simulink model "sampleModel206"  (R2021b)
settings: Solver=VariableStepAuto  StartTime=0.0  StopTime=10.0  RelTol=1e-3
libraries: simulink x9, slpidlib x1
settings Model: Creator=user  LastModifiedBy=user

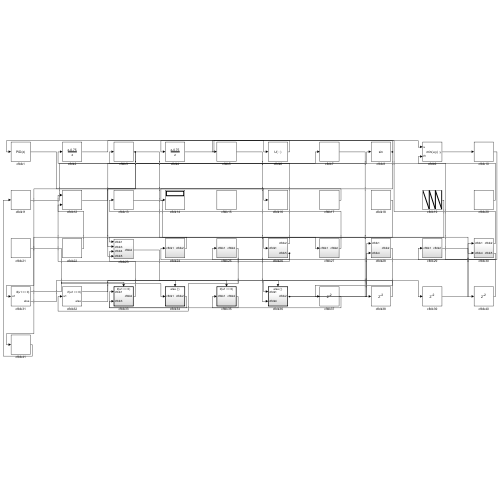
[thumbnail: Simulink's stored preview of the top-level diagram]
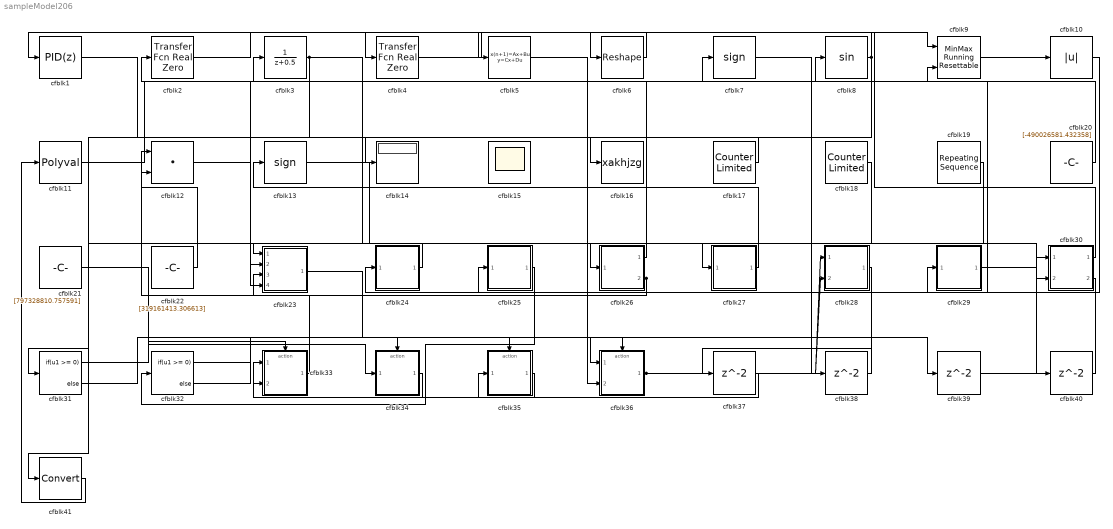
== system sampleModel206 ==
  cfblk1 : slpidlib/PID Controller  Controller=PID  Form=Parallel  TimeDomain=Discrete-time  UseExternalTs=off  SampleTime=1  IntegratorMethod=Forward Euler  FilterMethod=Forward Euler  ControllerParametersSource=internal  P=1  I=1  D=0  UseFilter=on  N=100  TunerSelectOption=Transfer Function Based (PID Tuner App)  InitialConditionSource=internal  InitialConditionForIntegrator=0  InitialConditionForFilter=0  DifferentiatorICPrevScaledInput=0  ExternalReset=none  TrackingMode=off  Kt=1  LimitOutput=off  SatLimitsSource=internal  UpperSaturationLimit=inf  LowerSaturationLimit=-inf  LinearizeAsGain=off  AntiWindupMode=none  Kb=1  POutMin=[]  POutMax=[]  IOutMin=[]  IOutMax=[]  DOutMin=[]  DOutMax=[]  NOutMin=[]  NOutMax=[]  SumOutMin=[]  SumOutMax=[]  SaturationOutMin=[]  SaturationOutMax=[]  PParamMin=[]  PParamMax=[]  IParamMin=[]  IParamMax=[]  DParamMin=[]  DParamMax=[]  NParamMin=[]  NParamMax=[]  KbParamMin=[]  KbParamMax=[]  KtParamMin=[]  KtParamMax=[]  KbOutMin=[]  KbOutMax=[]  KtOutMin=[]  KtOutMax=[]  IntegratorOutMin=[]  IntegratorOutMax=[]  FilterOutMin=[]  FilterOutMax=[]  SumI1OutMin=[]  SumI1OutMax=[]  SumI2OutMin=[]  SumI2OutMax=[]  SumI3OutMin=[]  SumI3OutMax=[]  SumI4OutMin=[]  SumI4OutMax=[]  SumDOutMin=[]  SumDOutMax=[]  DifferentiatorOutMin=[]  DifferentiatorOutMax=[]  FilterDiffOutCoefMin=[]  FilterDiffOutCoefMax=[]  ReciprocalOutMin=[]  ReciprocalOutMax=[]  SumDenOutMin=[]  SumDenOutMax=[]  SumNumOutMin=[]  SumNumOutMax=[]  DivideOutMin=[]  DivideOutMax=[]  UdiffTsProdOutMin=[]  UdiffTsProdOutMax=[]  NTsProdOutMin=[]  NTsProdOutMax=[]  UintegralTsProdOutMin=[]  UintegralTsProdOutMax=[]  UngainTsProdOutMin=[]  UngainTsProdOutMax=[]  IntegratorContinuousStateAttributes=''  IntegratorStateMustResolveToSignalObject=off  IntegratorRTWStateStorageClass=Auto  FilterContinuousStateAttributes=''  FilterStateMustResolveToSignalObject=off  FilterRTWStateStorageClass=Auto  ParallelPVariant=InternalParameters  IdealPVariant=Disabled  IVariant=InternalParameters  DVariant=InternalParameters  IntegratorVariant=Discrete  SatVariant=Disabled  AWVariant=Passthrough  PCopyVariant=Disabled  TRVariant=Disabled  FdbkBlocksVariant=Forward  IdealPFdbkVariant=Disabled  SatFdbkVariant=Disabled  DerivativeFilterVariant=ForwardEulerFilter  NVariant=InternalParameters  NCopyVariant=Disabled  FilterICVariant=InternalICsFilter  IntegratorICVariant=InternalICs  ExternalResetVariant=Disabled  TRSumVariant=Passthrough  SumFdbkVariant=Disabled  SumVariant=Sum_PID  TsampFilterVariant=InternalTs  TsampNgainVariant=Passthrough  TsampIntegralVariant=Passthrough  ExternalSaturationOutDataTypeStr=Inherit: Same as second input
  cfblk10 : Abs
  cfblk11 : Polyval  Coefs=[ +2.081618890e-019, -1.441693666e-014, +4.719686976e-010, -8.536869453e-006, +1.621573104e-001, -8.087801117e+001 ]
  cfblk12 : DotProduct  InputSameDT=on  OutDataTypeStr=Inherit: Inherit via internal rule
  cfblk13 : Signum
  cfblk14 : Display
  cfblk15 : Scope
      settings: Floating=on
  cfblk16 : ToWorkspace  VariableName=xakhjzg  SaveFormat=Timeseries  SampleTime=-1
  cfblk17 : simulink/Sources/Counter Limited  uplimit=[229.000000]  tsamp=-1
  cfblk18 : simulink/Sources/Counter Limited  uplimit=[557.000000]  tsamp=-1
  cfblk19 : simulink/Sources/Repeating Sequence  rep_seq_t=[0 2]  rep_seq_y=[57928011.441272, -161595305.218500]
  cfblk2 : simulink/Discrete/Transfer Fcn Real Zero  ZeroZ=0.75  ICPrevInput=0.0  DoSatur=off
      settings: SourceProductBaseCode=SL
  cfblk20 : Constant  Value=[-490026581.432358]  SampleTime=1
  cfblk21 : Constant  Value=[797328810.757591]  SampleTime=1
  cfblk22 : Constant  Value=[319161413.306613]  SampleTime=1
  cfblk23 : Subsystem
  cfblk24 : Subsystem
  cfblk25 : Subsystem
  cfblk26 : Subsystem
  cfblk27 : Subsystem
  cfblk28 : Subsystem
  cfblk29 : Subsystem
  cfblk3 : DiscreteTransferFcn  SampleTime=1
  cfblk30 : Subsystem
  cfblk31 : If  IfExpression=u1 >= 0  SampleTime=1
  cfblk32 : If  IfExpression=u1 >= 0  SampleTime=1
  cfblk33 : Subsystem  TreatAsAtomicUnit=on
  cfblk34 : Subsystem  TreatAsAtomicUnit=on
  cfblk35 : Subsystem  TreatAsAtomicUnit=on
  cfblk36 : Subsystem  TreatAsAtomicUnit=on
  cfblk{37..40} (4 alike) : Delay  SampleTime=1
  cfblk4 : simulink/Discrete/Transfer Fcn Real Zero  ZeroZ=0.75  ICPrevInput=0.0  DoSatur=off
      settings: SourceProductBaseCode=SL
  cfblk41 : DataTypeConversion
  cfblk5 : DiscreteStateSpace
  cfblk6 : Reshape
  cfblk7 : Signum
  cfblk8 : Trigonometry
  cfblk9 : simulink/Math Operations/MinMax Running Resettable  Function=min  vinit=0.0
  wires:
  cfblk11/1 -> cfblk8/1
  cfblk24/1(cfblk2) -> cfblk23/1(cfblk1)
  cfblk30/1(cfblk2) -> cfblk1/1
  cfblk27/1(cfblk2) -> cfblk13/1
  cfblk5/1 -> cfblk36/2(cfblk4)
  cfblk20/1 -> cfblk3/1
  cfblk4/1 -> cfblk9/1
  cfblk21/1 -> cfblk34/1(cfblk1)
  cfblk10/1 -> cfblk29/1(cfblk1)
  cfblk34/1(cfblk2) -> cfblk33/1(cfblk1)
  cfblk25/1(cfblk2) -> cfblk32/1
  cfblk9/1 -> cfblk10/1
  cfblk12/1 -> cfblk7/1
  cfblk8/1 -> cfblk4/1, cfblk31/1
  cfblk6/1 -> cfblk5/1
  cfblk19/1 -> cfblk26/1(cfblk1)
  cfblk13/1 -> cfblk30/2(cfblk4)
  cfblk35/1(cfblk2) -> cfblk33/2(cfblk3)
  cfblk33/1(cfblk2) -> cfblk12/1
  cfblk26/1(cfblk2) -> cfblk2/1
  cfblk26/2(cfblk5) -> cfblk25/1(cfblk1), cfblk23/3(cfblk4)
  cfblk17/1 -> cfblk14/1
  cfblk2/1 -> cfblk6/1
  cfblk22/1 -> cfblk12/2
  cfblk3/1 -> cfblk27/1(cfblk1), cfblk23/2(cfblk3), cfblk23/4(cfblk5)
  cfblk1/1 -> cfblk16/1
  cfblk36/1(cfblk2) -> cfblk28/1(cfblk1), cfblk28/2(cfblk4)
  cfblk30/2(cfblk5) -> cfblk24/1(cfblk1)
  cfblk31/1 -> cfblk33/Action
  cfblk31/2 -> cfblk34/Action
  cfblk32/1 -> cfblk35/Action
  cfblk32/2 -> cfblk36/Action
  cfblk28/1(cfblk2) -> cfblk37/1
  cfblk37/1 -> cfblk35/1(cfblk1)
  cfblk7/1 -> cfblk38/1
  cfblk38/1 -> cfblk36/1(cfblk1)
  cfblk23/1(cfblk2) -> cfblk39/1
  cfblk39/1 -> cfblk30/1(cfblk1)
  cfblk29/1(cfblk2) -> cfblk40/1
  cfblk40/1 -> cfblk9/2
  cfblk18/1 -> cfblk41/1
  cfblk41/1 -> cfblk11/1

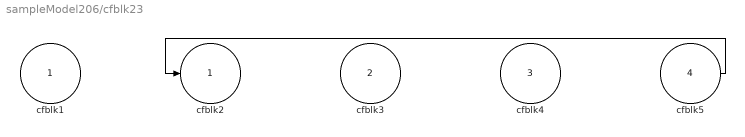
== system sampleModel206/cfblk23 ==
  cfblk1 : Inport
  cfblk3 : Inport  Port=2
  cfblk4 : Inport  Port=3
  cfblk5 : Inport  Port=4
  cfblk2 : Outport
  wires:
  cfblk5/1 -> cfblk2/1

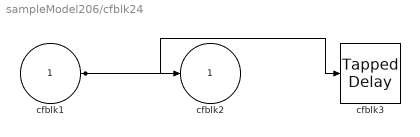
== system sampleModel206/cfblk24 ==
  cfblk1 : Inport
  cfblk3 : simulink/Discrete/Tapped Delay  vinit=0.0  samptime=-1  NumDelays=1  DelayOrder=Oldest  includeCurrent=off
  cfblk2 : Outport
  wires:
  cfblk1/1 -> cfblk2/1, cfblk3/1

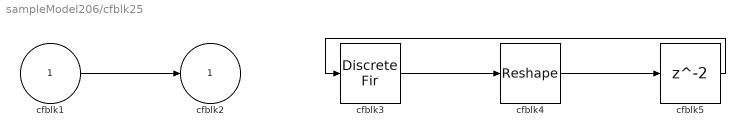
== system sampleModel206/cfblk25 ==
  cfblk1 : Inport
  cfblk3 : DiscreteFir  SampleTime=1
  cfblk4 : Reshape
  cfblk5 : Delay  SampleTime=1
  cfblk2 : Outport
  wires:
  cfblk1/1 -> cfblk2/1
  cfblk3/1 -> cfblk4/1
  cfblk4/1 -> cfblk5/1
  cfblk5/1 -> cfblk3/1

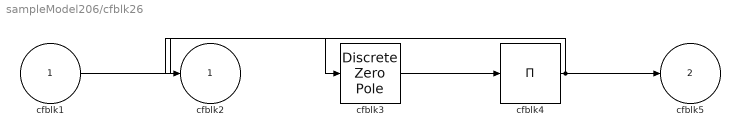
== system sampleModel206/cfblk26 ==
  cfblk1 : Inport
  cfblk3 : DiscreteZeroPole  Poles=[0 0.5]  Gain=1
  cfblk4 : Product  Inputs=*
  cfblk2 : Outport
  cfblk5 : Outport  Port=2
  wires:
  cfblk3/1 -> cfblk4/1
  cfblk4/1 -> cfblk5/1, cfblk2/1
  cfblk1/1 -> cfblk3/1

== system sampleModel206/cfblk27 ==
  cfblk1 : Inport
  cfblk3 : Bias  Bias=[-16445692.538380]
  cfblk2 : Outport
  wires:
  cfblk1/1 -> cfblk3/1
  cfblk3/1 -> cfblk2/1

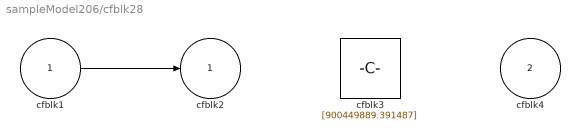
== system sampleModel206/cfblk28 ==
  cfblk1 : Inport
  cfblk4 : Inport  Port=2
  cfblk3 : Constant  Value=[900449889.391487]  SampleTime=1
  cfblk2 : Outport
  wires:
  cfblk1/1 -> cfblk2/1

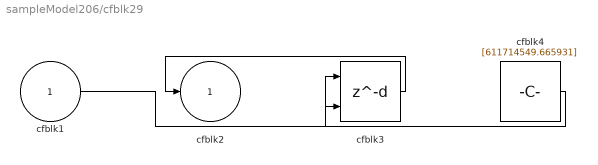
== system sampleModel206/cfblk29 ==
  cfblk1 : Inport
  cfblk3 : Delay  DelayLengthSource=Input port  SampleTime=1
      settings: InputPortMap=u0,p1
  cfblk4 : Constant  Value=[611714549.665931]  SampleTime=1
  cfblk2 : Outport
  wires:
  cfblk3/1 -> cfblk2/1
  cfblk1/1 -> cfblk3/1
  cfblk4/1 -> cfblk3/2

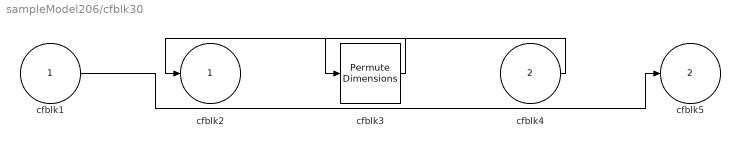
== system sampleModel206/cfblk30 ==
  cfblk1 : Inport
  cfblk4 : Inport  Port=2
  cfblk3 : PermuteDimensions
  cfblk2 : Outport
  cfblk5 : Outport  Port=2
  wires:
  cfblk3/1 -> cfblk2/1
  cfblk1/1 -> cfblk5/1
  cfblk4/1 -> cfblk3/1

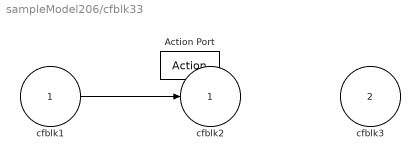
== system sampleModel206/cfblk33 ==
  cfblk1 : Inport
  cfblk3 : Inport  Port=2
  Action Port : ActionPort  ActionPortLabel=if(u1 >= 0)
  cfblk2 : Outport
  wires:
  cfblk1/1 -> cfblk2/1

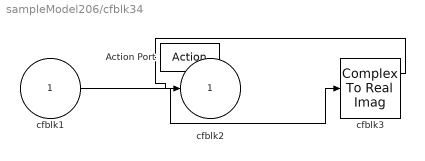
== system sampleModel206/cfblk34 ==
  cfblk1 : Inport
  Action Port : ActionPort  ActionPortLabel=else
  cfblk3 : ComplexToRealImag
  cfblk2 : Outport
  wires:
  cfblk1/1 -> cfblk3/1
  cfblk3/1 -> cfblk2/1

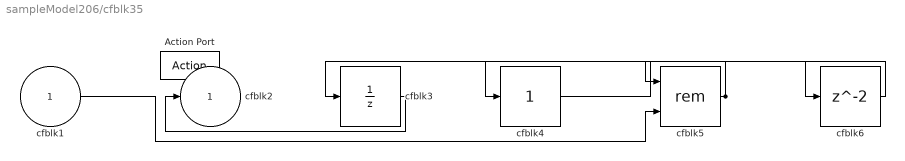
== system sampleModel206/cfblk35 ==
  cfblk1 : Inport
  Action Port : ActionPort  ActionPortLabel=if(u1 >= 0)
  cfblk3 : UnitDelay  SampleTime=-1  HasFrameUpgradeWarning=on
  cfblk4 : simulink/Math Operations/Slider Gain  gain=1  low=0  high=2
  cfblk5 : Math  Operator=rem  SaturateOnIntegerOverflow=on
  cfblk6 : Delay
  cfblk2 : Outport
  wires:
  cfblk3/1 -> cfblk2/1
  cfblk1/1 -> cfblk5/2
  cfblk5/1 -> cfblk4/1, cfblk3/1
  cfblk4/1 -> cfblk6/1
  cfblk6/1 -> cfblk5/1

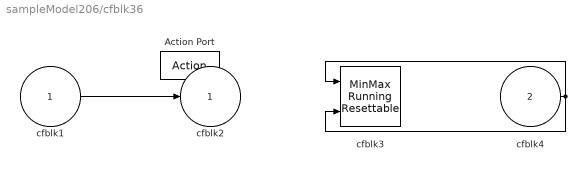
== system sampleModel206/cfblk36 ==
  cfblk1 : Inport
  cfblk4 : Inport  Port=2
  Action Port : ActionPort  ActionPortLabel=else
  cfblk3 : simulink/Math Operations/MinMax Running Resettable  Function=min  vinit=0.0
  cfblk2 : Outport
  wires:
  cfblk1/1 -> cfblk2/1
  cfblk4/1 -> cfblk3/1, cfblk3/2
